simulink model "SolarPanelTest"  (R2019a)
settings: Solver=VariableStepAuto  StartTime=0.0  StopTime=15*3600  RelTol=1e-3
undefined symbols (not defined in the file): J, Kd, Kf, Kg, Kt, L, R
libraries: simulink x1
settings Model: Creator=Safet  LastModifiedBy=Safet
settings DataIOCC: ExternalInput=[sunTime sunPosition]  LoadExternalInput=on

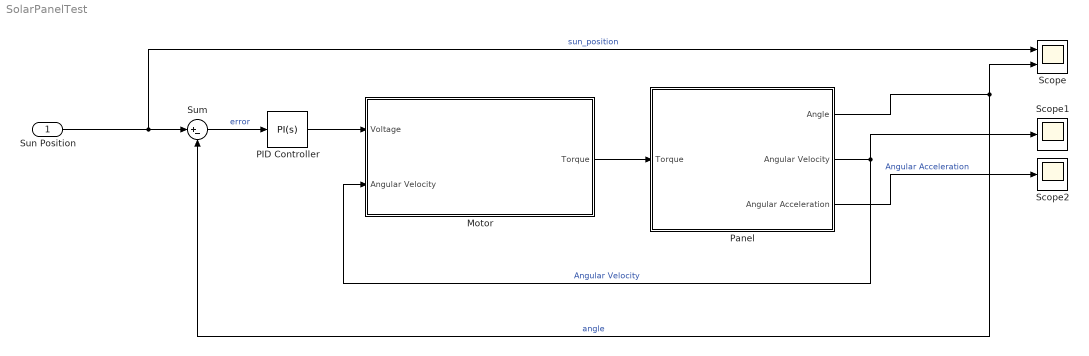
== system SolarPanelTest ==
  "Sun Position " : Inport
  Motor : Subsystem
  PID Controller : simulink/Continuous/PID Controller  Controller=PI  Form=Parallel  TimeDomain=Continuous-time  SampleTime=-1  IntegratorMethod=Forward Euler  FilterMethod=Forward Euler  ControllerParametersSource=internal  P=240  I=180  D=0  UseFilter=on  N=100  TunerSelectOption=Transfer Function Based (PID Tuner App)  InitialConditionSource=internal  InitialConditionForIntegrator=0  InitialConditionForFilter=0  DifferentiatorICPrevScaledInput=0  ExternalReset=none  TrackingMode=off  Kt=1  LimitOutput=off  UpperSaturationLimit=inf  LowerSaturationLimit=-inf  LinearizeAsGain=on  AntiWindupMode=none  Kb=1  POutMin=[]  POutMax=[]  IOutMin=[]  IOutMax=[]  DOutMin=[]  DOutMax=[]  NOutMin=[]  NOutMax=[]  SumOutMin=[]  SumOutMax=[]  SaturationOutMin=[]  SaturationOutMax=[]  PParamMin=[]  PParamMax=[]  IParamMin=[]  IParamMax=[]  DParamMin=[]  DParamMax=[]  NParamMin=[]  NParamMax=[]  KbParamMin=[]  KbParamMax=[]  KtParamMin=[]  KtParamMax=[]  KbOutMin=[]  KbOutMax=[]  KtOutMin=[]  KtOutMax=[]  IntegratorOutMin=[]  IntegratorOutMax=[]  FilterOutMin=[]  FilterOutMax=[]  SumI1OutMin=[]  SumI1OutMax=[]  SumI2OutMin=[]  SumI2OutMax=[]  SumI3OutMin=[]  SumI3OutMax=[]  SumI4OutMin=[]  SumI4OutMax=[]  SumDOutMin=[]  SumDOutMax=[]  DifferentiatorOutMin=[]  DifferentiatorOutMax=[]  FilterDiffOutCoefMin=[]  FilterDiffOutCoefMax=[]  ReciprocalOutMin=[]  ReciprocalOutMax=[]  SumDenOutMin=[]  SumDenOutMax=[]  SumNumOutMin=[]  SumNumOutMax=[]  DivideOutMin=[]  DivideOutMax=[]  IntegratorContinuousStateAttributes=''  IntegratorStateMustResolveToSignalObject=off  IntegratorRTWStateStorageClass=Auto  FilterContinuousStateAttributes=''  FilterStateMustResolveToSignalObject=off  FilterRTWStateStorageClass=Auto  ParallelPVariant=InternalParameters  IdealPVariant=Disabled  IVariant=InternalParameters  DVariant=Disabled  IntegratorVariant=Continuous  SatVariant=Disabled  AWVariant=Passthrough  PCopyVariant=Disabled  TRVariant=Disabled  FdbkBlocksVariant=Forward  IdealPFdbkVariant=Disabled  SatFdbkVariant=Disabled  DerivativeFilterVariant=Disabled  NVariant=Disabled  NCopyVariant=Disabled_SignalSpec  FilterICVariant=Disabled  IntegratorICVariant=InternalICs  ExternalResetVariant=Disabled  TRSumVariant=Passthrough  SumFdbkVariant=Disabled  SumVariant=Sum_PI
  Panel : Subsystem
  Scope : Scope  NumInputPorts=2
  Scope1 : Scope
  Scope2 : Scope
  Sum : Sum  Inputs=|+-
  wires:
  Panel/1(Angle) -> Sum/2, Scope/2  "angle"
  Panel/2(Angular Velocity) -> Scope1/1, Motor/2(Angular Velocity)  "Angular Velocity"
  Panel/3(Angular Acceleration) -> Scope2/1  "Angular Acceleration"
  Motor/1(Torque) -> Panel/1(Torque)
  "Sun Position "/1 -> Scope/1, Sum/1  "sun_position"
  Sum/1 -> PID Controller/1  "error"
  PID Controller/1 -> Motor/1(Voltage)

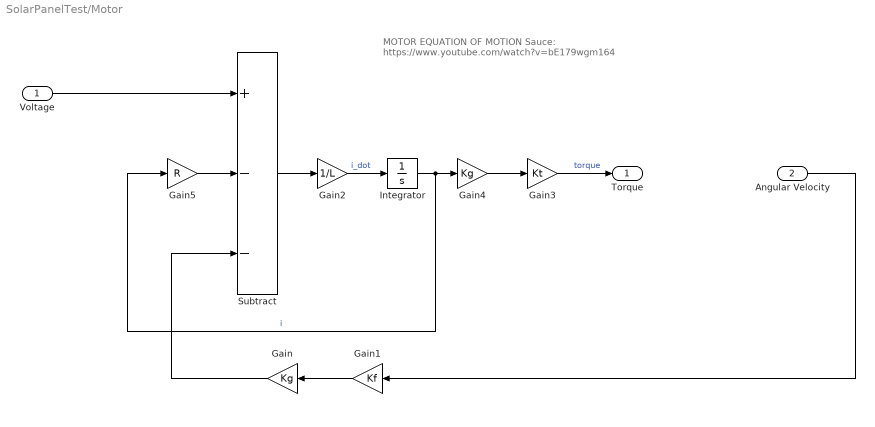
== system SolarPanelTest/Motor ==
  note: MOTOR EQUATION OF MOTION
      |
      | Sauce: https://www.youtube.com/watch?v=bE179wgm164
  Voltage : Inport
  Angular Velocity : Inport  Port=2
  Gain : Gain  Gain=Kg
  Gain1 : Gain  Gain=Kf
  Gain2 : Gain  Gain=1/L
  Gain3 : Gain  Gain=Kt
  Gain4 : Gain  Gain=Kg
  Gain5 : Gain  Gain=R
  Integrator : Integrator
  Subtract : Sum  Inputs=+--
  Torque : Outport
  wires:
  Integrator/1 -> Gain5/1, Gain4/1  "i"
  Gain4/1 -> Gain3/1
  Voltage/1 -> Subtract/1
  Gain/1 -> Subtract/3
  Gain5/1 -> Subtract/2
  Subtract/1 -> Gain2/1
  Gain2/1 -> Integrator/1  "i_dot"
  Gain1/1 -> Gain/1
  Angular Velocity/1 -> Gain1/1
  Gain3/1 -> Torque/1  "torque"

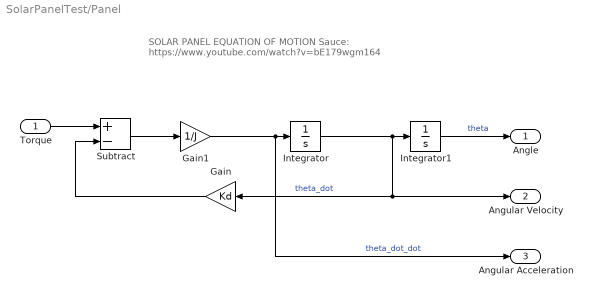
== system SolarPanelTest/Panel ==
  note: SOLAR PANEL EQUATION OF MOTION
      |
      | Sauce: https://www.youtube.com/watch?v=bE179wgm164
  Torque : Inport
  Gain : Gain  Gain=Kd
  Gain1 : Gain  Gain=1/J
  Integrator : Integrator
  Integrator1 : Integrator
  Subtract : Sum  Inputs=+-
  Angle : Outport
  Angular Velocity : Outport  Port=2
  Angular Acceleration : Outport  Port=3
  wires:
  Gain/1 -> Subtract/2
  Integrator/1 -> Angular Velocity/1, Gain/1, Integrator1/1  "theta_dot"
  Subtract/1 -> Gain1/1
  Integrator1/1 -> Angle/1  "theta"
  Gain1/1 -> Angular Acceleration/1, Integrator/1  "theta_dot_dot"
  Torque/1 -> Subtract/1
